simulink model "final_quadruped_040722_zmp"  (R2021a)
settings: Solver=ode15s  StartTime=0.0  StopTime=10  FixedStep=1e-3  RelTol=1e-5  EnableMultiTasking=on
values from neighbouring files (symbols this model uses):
  foot_x = 8    [bipedparameters.m]    (also in fcn.m; finalrobotParameters.m; finalrobotParameters_110522.m; finalrobotParameters_140522.m)
  foot_y = 6    [bipedparameters.m]    (also in fcn.m; finalrobotParameters.m; finalrobotParameters_110522.m; finalrobotParameters_140522.m)
  foot_z = 1    [bipedparameters.m]    (also in fcn.m; finalrobotParameters.m; finalrobotParameters_110522.m; finalrobotParameters_140522.m)
  height_plane = 0.025    [bipedparameters.m]    (also in finalrobotParameters.m; finalrobotParameters_110522.m; finalrobotParameters_140522.m; finalrobotParameters_240522.m)
  kd_ankle = 1000    [bipedparameters.m]    (also in finalrobotParameters_240522.m)
  kd_hip = 1000    [bipedparameters.m]    (also in finalrobotParameters_240522.m)
  kd_knee = 1000    [bipedparameters.m]    (also in finalrobotParameters_240522.m)
  ki_ankle = 1000    [bipedparameters.m]    (also in finalrobotParameters_240522.m)
  ki_hip = 1000    [bipedparameters.m]    (also in finalrobotParameters_240522.m)
  ki_knee = 2000    [bipedparameters.m]    (also in finalrobotParameters_240522.m)
  kp_ankle = 1000    [bipedparameters.m]    (also in finalrobotParameters_240522.m)
  kp_hip = 1000    [bipedparameters.m]    (also in finalrobotParameters_240522.m)
  kp_knee = 2000    [bipedparameters.m]    (also in finalrobotParameters_240522.m)
  lower_leg_length = 10    [bipedparameters.m]    (also in fcn.m; finalrobotParameters.m; finalrobotParameters_110522.m; finalrobotParameters_140522.m)
  plane_x = 25    [bipedparameters.m]    (also in finalrobotParameters.m; finalrobotParameters_110522.m; finalrobotParameters_140522.m; finalrobotParameters_240522.m)
  plane_y = 3    [bipedparameters.m]    (also in finalrobotParameters.m; finalrobotParameters_110522.m; finalrobotParameters_140522.m; finalrobotParameters_240522.m)
  torso_offset_x = -0.5    [bipedparameters.m]    (also in finalrobotParameters.m = 10; finalrobotParameters_110522.m = 10; finalrobotParameters_140522.m = 10; finalrobotParameters_240522.m = 10)
  torso_offset_z = -2    [bipedparameters.m]    (also in finalrobotParameters.m; finalrobotParameters_110522.m; finalrobotParameters_140522.m; finalrobotParameters_240522.m)
  torso_x = 5    [bipedparameters.m]    (also in fcn.m = 25; finalrobotParameters.m = 25; finalrobotParameters_110522.m = 25; finalrobotParameters_140522.m = 25)
  torso_y = 10    [bipedparameters.m]    (also in fcn.m = 16; finalrobotParameters.m = 16; finalrobotParameters_110522.m = 16; finalrobotParameters_140522.m = 16)
  torso_z = 8    [bipedparameters.m]    (also in fcn.m = 10; finalrobotParameters.m = 10; finalrobotParameters_110522.m = 10; finalrobotParameters_140522.m = 10)
  upper_leg_length = 10    [bipedparameters.m]    (also in fcn.m; finalrobotParameters.m; finalrobotParameters_110522.m; finalrobotParameters_140522.m)
undefined symbols (not defined in the file or in its folder): sigbuilder_block, X, Y, Z
libraries: nesl_utility x288, sm_lib x71, pid_lib x20, Contact_Forces_Lib x16, fl_lib x3
(part 8 of 9)

== system final_quadruped_040722_zmp/Model/Right Leg Front /Hip ==
  note: accelerationRFhip
  t2ddhip : Inport
  tddRF_hip : Inport  Port=2
  Gimbal Joint : sm_lib/Joints/Gimbal Joint  JointMode=Normal  SenseConstraintForce=off  SenseConstraintForceX=off  SenseConstraintForceY=off  SenseConstraintForceZ=off  SenseConstraintTorque=off  SenseConstraintTorqueX=off  SenseConstraintTorqueY=off  SenseConstraintTorqueZ=off  SenseTotalForce=off  SenseTotalForceX=off  SenseTotalForceY=off  SenseTotalForceZ=off  SenseTotalTorque=off  SenseTotalTorqueX=off  SenseTotalTorqueY=off  SenseTotalTorqueZ=off  CompositeWrenchDir=FollowerOnBase  CompositeWrenchFrame=BaseFrame  RxEquilibriumPosition=0  RxEquilibriumPositionUnits=deg  RxSpringStiffness=0  RxSpringStiffnessUnits=N*m/deg  RxDampingCoefficient=0  RxDampingCoefficientUnits=N*m/(deg/s)  RxTorqueActuationMode=InputTorque  RxMotionActuationMode=ComputedMotion  RxSensePosition=on  RxSenseVelocity=on  RxSenseAcceleration=on  RxSenseTorqueForce=off  RxSenseLowerLimitTorqueForce=off  RxSenseUpperLimitTorqueForce=off  RxLowerLimitSpecify=off  RxLowerLimitBound=-90  RxLowerLimitBoundUnits=deg  RxLowerLimitStiffness=1e4  RxLowerLimitStiffnessUnits=N*m/deg  RxLowerLimitDamping=10  RxLowerLimitDampingUnits=N*m/(deg/s)  RxLowerLimitTransitionRegionWidth=0.1  RxLowerLimitTransitionRegionWidthUnits=deg  RxUpperLimitSpecify=off  RxUpperLimitBound=90  RxUpperLimitBoundUnits=deg  RxUpperLimitStiffness=1e4  RxUpperLimitStiffnessUnits=N*m/deg  RxUpperLimitDamping=10  RxUpperLimitDampingUnits=N*m/(deg/s)  RxUpperLimitTransitionRegionWidth=0.1  RxUpperLimitTransitionRegionWidthUnits=deg  RxPositionTargetSpecify=off  RxPositionTargetPriority=High  RxPositionTargetValue=0  RxPositionTargetValueUnits=deg  RxVelocityTargetSpecify=off  RxVelocityTargetPriority=High  RxVelocityTargetValue=0  RxVelocityTargetValueUnits=deg/s  RyEquilibriumPosition=0  RyEquilibriumPositionUnits=deg  RySpringStiffness=0  RySpringStiffnessUnits=N*m/deg  RyDampingCoefficient=0  RyDampingCoefficientUnits=N*m/(deg/s)  RyTorqueActuationMode=InputTorque  RyMotionActuationMode=ComputedMotion  RySensePosition=on  RySenseVelocity=on  RySenseAcceleration=on  RySenseTorqueForce=off  RySenseLowerLimitTorqueForce=off  RySenseUpperLimitTorqueForce=off  RyLowerLimitSpecify=off  RyLowerLimitBound=-90  RyLowerLimitBoundUnits=deg  RyLowerLimitStiffness=1e4  RyLowerLimitStiffnessUnits=N*m/deg  RyLowerLimitDamping=10  RyLowerLimitDampingUnits=N*m/(deg/s)  RyLowerLimitTransitionRegionWidth=0.1  RyLowerLimitTransitionRegionWidthUnits=deg  RyUpperLimitSpecify=off  RyUpperLimitBound=90  RyUpperLimitBoundUnits=deg  RyUpperLimitStiffness=1e4  RyUpperLimitStiffnessUnits=N*m/deg  RyUpperLimitDamping=10  RyUpperLimitDampingUnits=N*m/(deg/s)  RyUpperLimitTransitionRegionWidth=0.1  RyUpperLimitTransitionRegionWidthUnits=deg  RyPositionTargetSpecify=off  RyPositionTargetPriority=High  RyPositionTargetValue=0  RyPositionTargetValueUnits=deg  RyVelocityTargetSpecify=off  RyVelocityTargetPriority=High  RyVelocityTargetValue=0  RyVelocityTargetValueUnits=deg/s  RzEquilibriumPosition=0  RzEquilibriumPositionUnits=deg  RzSpringStiffness=0  RzSpringStiffnessUnits=N*m/deg  RzDampingCoefficient=0  RzDampingCoefficientUnits=N*m/(deg/s)  RzTorqueActuationMode=InputTorque  RzMotionActuationMode=ComputedMotion  RzSensePosition=on  RzSenseVelocity=on  RzSenseAcceleration=on  RzSenseTorqueForce=off  RzSenseLowerLimitTorqueForce=off  RzSenseUpperLimitTorqueForce=off  RzLowerLimitSpecify=off  RzLowerLimitBound=-90  RzLowerLimitBoundUnits=deg  RzLowerLimitStiffness=1e4  RzLowerLimitStiffnessUnits=N*m/deg  RzLowerLimitDamping=10  RzLowerLimitDampingUnits=N*m/(deg/s)  RzLowerLimitTransitionRegionWidth=0.1  RzLowerLimitTransitionRegionWidthUnits=deg  RzUpperLimitSpecify=off  RzUpperLimitBound=90  RzUpperLimitBoundUnits=deg  RzUpperLimitStiffness=1e4  RzUpperLimitStiffnessUnits=N*m/deg  RzUpperLimitDamping=10  RzUpperLimitDampingUnits=N*m/(deg/s)  RzUpperLimitTransitionRegionWidth=0.1  RzUpperLimitTransitionRegionWidthUnits=deg  RzPositionTargetSpecify=on  RzPositionTargetPriority=Low  RzPositionTargetValue=-13  RzPositionTargetValueUnits=deg  RzVelocityTargetSpecify=on  RzVelocityTargetPriority=Low  RzVelocityTargetValue=1  RzVelocityTargetValueUnits=deg/s
  MATLAB Function : MATLAB Function  TreatAsAtomicUnit=on
  MATLAB Function1 : MATLAB Function  TreatAsAtomicUnit=on
  MATLAB Function2 : MATLAB Function  TreatAsAtomicUnit=on
  MATLAB Function3 : MATLAB Function  TreatAsAtomicUnit=on
  PID Controller : pid_lib/PID Controller  Controller=PID  Form=Parallel  TimeDomain=Continuous-time  UseExternalTs=off  SampleTime=-1  IntegratorMethod=Forward Euler  FilterMethod=Forward Euler  ControllerParametersSource=internal  P=kp_hip  I=ki_hip  D=kd_hip  UseFilter=on  N=100  TunerSelectOption=Transfer Function Based (PID Tuner App)  InitialConditionSource=internal  InitialConditionForIntegrator=0  InitialConditionForFilter=0  DifferentiatorICPrevScaledInput=0  ExternalReset=none  TrackingMode=off  Kt=1  LimitOutput=off  SatLimitsSource=internal  UpperSaturationLimit=inf  LowerSaturationLimit=-inf  LinearizeAsGain=on  AntiWindupMode=none  Kb=1  POutMin=[]  POutMax=[]  IOutMin=[]  IOutMax=[]  DOutMin=[]  DOutMax=[]  NOutMin=[]  NOutMax=[]  SumOutMin=[]  SumOutMax=[]  SaturationOutMin=[]  SaturationOutMax=[]  PParamMin=[]  PParamMax=[]  IParamMin=[]  IParamMax=[]  DParamMin=[]  DParamMax=[]  NParamMin=[]  NParamMax=[]  KbParamMin=[]  KbParamMax=[]  KtParamMin=[]  KtParamMax=[]  KbOutMin=[]  KbOutMax=[]  KtOutMin=[]  KtOutMax=[]  IntegratorOutMin=[]  IntegratorOutMax=[]  FilterOutMin=[]  FilterOutMax=[]  SumI1OutMin=[]  SumI1OutMax=[]  SumI2OutMin=[]  SumI2OutMax=[]  SumI3OutMin=[]  SumI3OutMax=[]  SumI4OutMin=[]  SumI4OutMax=[]  SumDOutMin=[]  SumDOutMax=[]  DifferentiatorOutMin=[]  DifferentiatorOutMax=[]  FilterDiffOutCoefMin=[]  FilterDiffOutCoefMax=[]  ReciprocalOutMin=[]  ReciprocalOutMax=[]  SumDenOutMin=[]  SumDenOutMax=[]  SumNumOutMin=[]  SumNumOutMax=[]  DivideOutMin=[]  DivideOutMax=[]  UdiffTsProdOutMin=[]  UdiffTsProdOutMax=[]  NTsProdOutMin=[]  NTsProdOutMax=[]  UintegralTsProdOutMin=[]  UintegralTsProdOutMax=[]  UngainTsProdOutMin=[]  UngainTsProdOutMax=[]  IntegratorContinuousStateAttributes=''  IntegratorStateMustResolveToSignalObject=off  IntegratorRTWStateStorageClass=Auto  FilterContinuousStateAttributes=''  FilterStateMustResolveToSignalObject=off  FilterRTWStateStorageClass=Auto  ParallelPVariant=InternalParameters  IdealPVariant=Disabled  IVariant=InternalParameters  DVariant=InternalParameters  IntegratorVariant=Continuous  SatVariant=Disabled  AWVariant=Passthrough  PCopyVariant=Disabled  TRVariant=Disabled  FdbkBlocksVariant=Forward  IdealPFdbkVariant=Disabled  SatFdbkVariant=Disabled  DerivativeFilterVariant=ContFilter  NVariant=InternalParameters  NCopyVariant=Disabled  FilterICVariant=InternalICsFilter  IntegratorICVariant=InternalICs  ExternalResetVariant=Disabled  TRSumVariant=Passthrough  SumFdbkVariant=Disabled  SumVariant=Sum_PID  TsampFilterVariant=InternalTs  TsampNgainVariant=Passthrough  TsampIntegralVariant=Passthrough  ExternalSaturationOutDataTypeStr=Inherit: Same as second input
  PID Controller1 : pid_lib/PID Controller  Controller=PID  Form=Parallel  TimeDomain=Continuous-time  UseExternalTs=off  SampleTime=-1  IntegratorMethod=Forward Euler  FilterMethod=Forward Euler  ControllerParametersSource=internal  P=kp_hip  I=ki_hip  D=kd_hip  UseFilter=on  N=100  TunerSelectOption=Transfer Function Based (PID Tuner App)  InitialConditionSource=internal  InitialConditionForIntegrator=0  InitialConditionForFilter=0  DifferentiatorICPrevScaledInput=0  ExternalReset=none  TrackingMode=off  Kt=1  LimitOutput=off  SatLimitsSource=internal  UpperSaturationLimit=inf  LowerSaturationLimit=-inf  LinearizeAsGain=on  AntiWindupMode=none  Kb=1  POutMin=[]  POutMax=[]  IOutMin=[]  IOutMax=[]  DOutMin=[]  DOutMax=[]  NOutMin=[]  NOutMax=[]  SumOutMin=[]  SumOutMax=[]  SaturationOutMin=[]  SaturationOutMax=[]  PParamMin=[]  PParamMax=[]  IParamMin=[]  IParamMax=[]  DParamMin=[]  DParamMax=[]  NParamMin=[]  NParamMax=[]  KbParamMin=[]  KbParamMax=[]  KtParamMin=[]  KtParamMax=[]  KbOutMin=[]  KbOutMax=[]  KtOutMin=[]  KtOutMax=[]  IntegratorOutMin=[]  IntegratorOutMax=[]  FilterOutMin=[]  FilterOutMax=[]  SumI1OutMin=[]  SumI1OutMax=[]  SumI2OutMin=[]  SumI2OutMax=[]  SumI3OutMin=[]  SumI3OutMax=[]  SumI4OutMin=[]  SumI4OutMax=[]  SumDOutMin=[]  SumDOutMax=[]  DifferentiatorOutMin=[]  DifferentiatorOutMax=[]  FilterDiffOutCoefMin=[]  FilterDiffOutCoefMax=[]  ReciprocalOutMin=[]  ReciprocalOutMax=[]  SumDenOutMin=[]  SumDenOutMax=[]  SumNumOutMin=[]  SumNumOutMax=[]  DivideOutMin=[]  DivideOutMax=[]  UdiffTsProdOutMin=[]  UdiffTsProdOutMax=[]  NTsProdOutMin=[]  NTsProdOutMax=[]  UintegralTsProdOutMin=[]  UintegralTsProdOutMax=[]  UngainTsProdOutMin=[]  UngainTsProdOutMax=[]  IntegratorContinuousStateAttributes=''  IntegratorStateMustResolveToSignalObject=off  IntegratorRTWStateStorageClass=Auto  FilterContinuousStateAttributes=''  FilterStateMustResolveToSignalObject=off  FilterRTWStateStorageClass=Auto  ParallelPVariant=InternalParameters  IdealPVariant=Disabled  IVariant=InternalParameters  DVariant=InternalParameters  IntegratorVariant=Continuous  SatVariant=Disabled  AWVariant=Passthrough  PCopyVariant=Disabled  TRVariant=Disabled  FdbkBlocksVariant=Forward  IdealPFdbkVariant=Disabled  SatFdbkVariant=Disabled  DerivativeFilterVariant=ContFilter  NVariant=InternalParameters  NCopyVariant=Disabled  FilterICVariant=InternalICsFilter  IntegratorICVariant=InternalICs  ExternalResetVariant=Disabled  TRSumVariant=Passthrough  SumFdbkVariant=Disabled  SumVariant=Sum_PID  TsampFilterVariant=InternalTs  TsampNgainVariant=Passthrough  TsampIntegralVariant=Passthrough  ExternalSaturationOutDataTypeStr=Inherit: Same as second input
  PID Controller2 : pid_lib/PID Controller  Controller=PID  Form=Parallel  TimeDomain=Continuous-time  UseExternalTs=off  SampleTime=-1  IntegratorMethod=Forward Euler  FilterMethod=Forward Euler  ControllerParametersSource=internal  P=kp_hip  I=ki_hip  D=kd_hip  UseFilter=on  N=100  TunerSelectOption=Transfer Function Based (PID Tuner App)  InitialConditionSource=internal  InitialConditionForIntegrator=0  InitialConditionForFilter=0  DifferentiatorICPrevScaledInput=0  ExternalReset=none  TrackingMode=off  Kt=1  LimitOutput=off  SatLimitsSource=internal  UpperSaturationLimit=inf  LowerSaturationLimit=-inf  LinearizeAsGain=on  AntiWindupMode=none  Kb=1  POutMin=[]  POutMax=[]  IOutMin=[]  IOutMax=[]  DOutMin=[]  DOutMax=[]  NOutMin=[]  NOutMax=[]  SumOutMin=[]  SumOutMax=[]  SaturationOutMin=[]  SaturationOutMax=[]  PParamMin=[]  PParamMax=[]  IParamMin=[]  IParamMax=[]  DParamMin=[]  DParamMax=[]  NParamMin=[]  NParamMax=[]  KbParamMin=[]  KbParamMax=[]  KtParamMin=[]  KtParamMax=[]  KbOutMin=[]  KbOutMax=[]  KtOutMin=[]  KtOutMax=[]  IntegratorOutMin=[]  IntegratorOutMax=[]  FilterOutMin=[]  FilterOutMax=[]  SumI1OutMin=[]  SumI1OutMax=[]  SumI2OutMin=[]  SumI2OutMax=[]  SumI3OutMin=[]  SumI3OutMax=[]  SumI4OutMin=[]  SumI4OutMax=[]  SumDOutMin=[]  SumDOutMax=[]  DifferentiatorOutMin=[]  DifferentiatorOutMax=[]  FilterDiffOutCoefMin=[]  FilterDiffOutCoefMax=[]  ReciprocalOutMin=[]  ReciprocalOutMax=[]  SumDenOutMin=[]  SumDenOutMax=[]  SumNumOutMin=[]  SumNumOutMax=[]  DivideOutMin=[]  DivideOutMax=[]  UdiffTsProdOutMin=[]  UdiffTsProdOutMax=[]  NTsProdOutMin=[]  NTsProdOutMax=[]  UintegralTsProdOutMin=[]  UintegralTsProdOutMax=[]  UngainTsProdOutMin=[]  UngainTsProdOutMax=[]  IntegratorContinuousStateAttributes=''  IntegratorStateMustResolveToSignalObject=off  IntegratorRTWStateStorageClass=Auto  FilterContinuousStateAttributes=''  FilterStateMustResolveToSignalObject=off  FilterRTWStateStorageClass=Auto  ParallelPVariant=InternalParameters  IdealPVariant=Disabled  IVariant=InternalParameters  DVariant=InternalParameters  IntegratorVariant=Continuous  SatVariant=Disabled  AWVariant=Passthrough  PCopyVariant=Disabled  TRVariant=Disabled  FdbkBlocksVariant=Forward  IdealPFdbkVariant=Disabled  SatFdbkVariant=Disabled  DerivativeFilterVariant=ContFilter  NVariant=InternalParameters  NCopyVariant=Disabled  FilterICVariant=InternalICsFilter  IntegratorICVariant=InternalICs  ExternalResetVariant=Disabled  TRSumVariant=Passthrough  SumFdbkVariant=Disabled  SumVariant=Sum_PID  TsampFilterVariant=InternalTs  TsampNgainVariant=Passthrough  TsampIntegralVariant=Passthrough  ExternalSaturationOutDataTypeStr=Inherit: Same as second input
  PS-Simulink Converter{,2..11} (11 alike) : nesl_utility/PS-Simulink Converter  PhysicalDomain=network_engine_domain  SubClassName=ps_output  LeftPortType=input  RightPortType=output  PseudoPeriodic=off  Frequencies=[]  Unit=inherit  AffineConversion=off
      settings: SourceProductBaseCode=PW,SS
  PS-Simulink Converter1 : nesl_utility/PS-Simulink Converter  PhysicalDomain=network_engine_domain  SubClassName=ps_output  LeftPortType=input  RightPortType=output  PseudoPeriodic=off  Frequencies=[]  Unit=1  AffineConversion=off
      settings: SourceProductBaseCode=PW,SS
  Scope{,1..6} (7 alike) : Scope
  Simulink-PS Converter : nesl_utility/Simulink-PS Converter  PhysicalDomain=network_engine_domain  SubClassName=ps_input  LeftPortType=input  RightPortType=output  PseudoPeriodic=off  Frequencies=[]  NoiseDistribution=none  NoiseParameters=[]  Unit=1  AffineConversion=off  FilteringAndDerivatives=provide  SimscapeFilterOrder=1  InputFilterTimeConstant=0.001  UdotUserProvided=0
      settings: SourceProductBaseCode=PW,SS
  Simulink-PS Converter1 : nesl_utility/Simulink-PS Converter  PhysicalDomain=network_engine_domain  SubClassName=ps_input  LeftPortType=input  RightPortType=output  PseudoPeriodic=off  Frequencies=[]  NoiseDistribution=none  NoiseParameters=[]  Unit=1  AffineConversion=off  FilteringAndDerivatives=provide  SimscapeFilterOrder=1  InputFilterTimeConstant=0.001  UdotUserProvided=0
      settings: SourceProductBaseCode=PW,SS
  Simulink-PS Converter2 : nesl_utility/Simulink-PS Converter  PhysicalDomain=network_engine_domain  SubClassName=ps_input  LeftPortType=input  RightPortType=output  PseudoPeriodic=off  Frequencies=[]  NoiseDistribution=none  NoiseParameters=[]  Unit=1  AffineConversion=off  FilteringAndDerivatives=provide  SimscapeFilterOrder=1  InputFilterTimeConstant=0.001  UdotUserProvided=0
      settings: SourceProductBaseCode=PW,SS
  Sum : Sum  Inputs=|+-
  Sum1 : Sum  Inputs=|+-
  Sum2 : Sum  Inputs=|+-
  Conn1 : PMIOPort  Side=Left
  Conn2 : PMIOPort  Port=2  Side=Right
  qx : PMIOPort  Port=3  Side=Right
  qy : PMIOPort  Port=4  Side=Right
  qz : PMIOPort  Port=5  Side=Right
  Outport2 : Outport
  Outport1 : Outport  Port=2
  Outport : Outport  Port=3
  wires:
  PS-Simulink Converter1/1 -> Sum/2  "speedRFhip"
  Sum/1 -> PID Controller/1, Scope/1
  PID Controller/1 -> Scope1/1, Simulink-PS Converter/1  "torqueRFhip"
  MATLAB Function1/1(hip) -> Outport2/1
  t2ddhip/1 -> Scope2/1
  PS-Simulink Converter/1 -> MATLAB Function/1(qx)
  PS-Simulink Converter4/1 -> MATLAB Function/2(qy)
  PS-Simulink Converter5/1 -> MATLAB Function/3(qz)
  MATLAB Function/1(hip) -> Outport1/1
  PS-Simulink Converter6/1 -> MATLAB Function1/1(wx)
  PS-Simulink Converter7/1 -> MATLAB Function1/2(wy)
  PS-Simulink Converter8/1 -> MATLAB Function1/3(wz)
  tddRF_hip/1 -> MATLAB Function2/1(tddRF)
  PID Controller1/1 -> Simulink-PS Converter1/1, Scope4/1  "torqueRFhip"
  Sum1/1 -> PID Controller1/1, Scope3/1
  MATLAB Function2/1(tddRFx) -> Sum1/1
  PS-Simulink Converter2/1 -> Sum1/2
  MATLAB Function2/3(tddRFz) -> Sum/1
  PID Controller2/1 -> Simulink-PS Converter2/1, Scope6/1  "torqueRFhip"
  Sum2/1 -> PID Controller2/1, Scope5/1
  MATLAB Function2/2(tddRFy) -> Sum2/1
  PS-Simulink Converter9/1 -> Sum2/2
  PS-Simulink Converter10/1 -> MATLAB Function3/1(bx)
  PS-Simulink Converter3/1 -> MATLAB Function3/3(bz)
  PS-Simulink Converter11/1 -> MATLAB Function3/2(by)
  MATLAB Function3/1(hip) -> Outport/1
  connections:
  Conn2/RConn1 -- Gimbal Joint/RConn1
  Conn1/RConn1 -- Gimbal Joint/LConn1
  Gimbal Joint/RConn2 -- qx/RConn1 -- PS-Simulink Converter/LConn1
  PS-Simulink Converter4/LConn1 -- Gimbal Joint/RConn5 -- qy/RConn1
  PS-Simulink Converter5/LConn1 -- Gimbal Joint/RConn8 -- qz/RConn1
  Gimbal Joint/RConn3 -- PS-Simulink Converter2/LConn1 -- PS-Simulink Converter6/LConn1
  PS-Simulink Converter7/LConn1 -- Gimbal Joint/RConn6 -- PS-Simulink Converter9/LConn1
  PS-Simulink Converter8/LConn1 -- Gimbal Joint/RConn9 -- PS-Simulink Converter1/LConn1
  Simulink-PS Converter1/RConn1 -- Gimbal Joint/LConn2
  Simulink-PS Converter2/RConn1 -- Gimbal Joint/LConn3
  Simulink-PS Converter/RConn1 -- Gimbal Joint/LConn4
  Gimbal Joint/RConn4 -- PS-Simulink Converter10/LConn1
  Gimbal Joint/RConn7 -- PS-Simulink Converter11/LConn1
  Gimbal Joint/RConn10 -- PS-Simulink Converter3/LConn1

== system final_quadruped_040722_zmp/Model/Right Leg Front /Knee ==
  note: accelerationRFknee
  note: Meas for knee
  tddRF_knee : Inport
  t2ddknee : Inport  Port=2
  Bus Creator : BusCreator  Inputs=3
  Knee joint : sm_lib/Joints/Revolute Joint  JointMode=Normal  SenseConstraintForce=off  SenseConstraintForceX=off  SenseConstraintForceY=off  SenseConstraintForceZ=off  SenseConstraintTorque=off  SenseConstraintTorqueX=off  SenseConstraintTorqueY=off  SenseConstraintTorqueZ=off  SenseTotalForce=off  SenseTotalForceX=off  SenseTotalForceY=off  SenseTotalForceZ=off  SenseTotalTorque=off  SenseTotalTorqueX=off  SenseTotalTorqueY=off  SenseTotalTorqueZ=off  CompositeWrenchDir=FollowerOnBase  CompositeWrenchFrame=BaseFrame  EquilibriumPosition=0  EquilibriumPositionUnits=deg  SpringStiffness=0  SpringStiffnessUnits=N*m/deg  DampingCoefficient=0  DampingCoefficientUnits=N*m/(deg/s)  TorqueActuationMode=InputTorque  MotionActuationMode=ComputedMotion  SensePosition=on  SenseVelocity=on  SenseAcceleration=on  SenseTorqueForce=off  SenseLowerLimitTorqueForce=off  SenseUpperLimitTorqueForce=off  LowerLimitSpecify=on  LowerLimitBound=0  LowerLimitBoundUnits=deg  LowerLimitStiffness=1e4  LowerLimitStiffnessUnits=N*m/deg  LowerLimitDamping=10  LowerLimitDampingUnits=N*m/(deg/s)  LowerLimitTransitionRegionWidth=0.1  LowerLimitTransitionRegionWidthUnits=deg  UpperLimitSpecify=on  UpperLimitBound=20  UpperLimitBoundUnits=deg  UpperLimitStiffness=1e4  UpperLimitStiffnessUnits=N*m/deg  UpperLimitDamping=10  UpperLimitDampingUnits=N*m/(deg/s)  UpperLimitTransitionRegionWidth=0.1  UpperLimitTransitionRegionWidthUnits=deg  PositionTargetSpecify=on  PositionTargetPriority=Low  PositionTargetValue=28  PositionTargetValueUnits=deg  VelocityTargetSpecify=on  VelocityTargetPriority=Low  VelocityTargetValue=-2  VelocityTargetValueUnits=deg/s
  PID Controller : pid_lib/PID Controller  Controller=PID  Form=Parallel  TimeDomain=Continuous-time  UseExternalTs=off  SampleTime=-1  IntegratorMethod=Forward Euler  FilterMethod=Forward Euler  ControllerParametersSource=internal  P=kp_knee  I=ki_knee  D=kd_knee  UseFilter=on  N=100  TunerSelectOption=Transfer Function Based (PID Tuner App)  InitialConditionSource=internal  InitialConditionForIntegrator=0  InitialConditionForFilter=0  DifferentiatorICPrevScaledInput=0  ExternalReset=none  TrackingMode=off  Kt=1  LimitOutput=off  SatLimitsSource=internal  UpperSaturationLimit=inf  LowerSaturationLimit=-inf  LinearizeAsGain=on  AntiWindupMode=none  Kb=1  POutMin=[]  POutMax=[]  IOutMin=[]  IOutMax=[]  DOutMin=[]  DOutMax=[]  NOutMin=[]  NOutMax=[]  SumOutMin=[]  SumOutMax=[]  SaturationOutMin=[]  SaturationOutMax=[]  PParamMin=[]  PParamMax=[]  IParamMin=[]  IParamMax=[]  DParamMin=[]  DParamMax=[]  NParamMin=[]  NParamMax=[]  KbParamMin=[]  KbParamMax=[]  KtParamMin=[]  KtParamMax=[]  KbOutMin=[]  KbOutMax=[]  KtOutMin=[]  KtOutMax=[]  IntegratorOutMin=[]  IntegratorOutMax=[]  FilterOutMin=[]  FilterOutMax=[]  SumI1OutMin=[]  SumI1OutMax=[]  SumI2OutMin=[]  SumI2OutMax=[]  SumI3OutMin=[]  SumI3OutMax=[]  SumI4OutMin=[]  SumI4OutMax=[]  SumDOutMin=[]  SumDOutMax=[]  DifferentiatorOutMin=[]  DifferentiatorOutMax=[]  FilterDiffOutCoefMin=[]  FilterDiffOutCoefMax=[]  ReciprocalOutMin=[]  ReciprocalOutMax=[]  SumDenOutMin=[]  SumDenOutMax=[]  SumNumOutMin=[]  SumNumOutMax=[]  DivideOutMin=[]  DivideOutMax=[]  UdiffTsProdOutMin=[]  UdiffTsProdOutMax=[]  NTsProdOutMin=[]  NTsProdOutMax=[]  UintegralTsProdOutMin=[]  UintegralTsProdOutMax=[]  UngainTsProdOutMin=[]  UngainTsProdOutMax=[]  IntegratorContinuousStateAttributes=''  IntegratorStateMustResolveToSignalObject=off  IntegratorRTWStateStorageClass=Auto  FilterContinuousStateAttributes=''  FilterStateMustResolveToSignalObject=off  FilterRTWStateStorageClass=Auto  ParallelPVariant=InternalParameters  IdealPVariant=Disabled  IVariant=InternalParameters  DVariant=InternalParameters  IntegratorVariant=Continuous  SatVariant=Disabled  AWVariant=Passthrough  PCopyVariant=Disabled  TRVariant=Disabled  FdbkBlocksVariant=Forward  IdealPFdbkVariant=Disabled  SatFdbkVariant=Disabled  DerivativeFilterVariant=ContFilter  NVariant=InternalParameters  NCopyVariant=Disabled  FilterICVariant=InternalICsFilter  IntegratorICVariant=InternalICs  ExternalResetVariant=Disabled  TRSumVariant=Passthrough  SumFdbkVariant=Disabled  SumVariant=Sum_PID  TsampFilterVariant=InternalTs  TsampNgainVariant=Passthrough  TsampIntegralVariant=Passthrough  ExternalSaturationOutDataTypeStr=Inherit: Same as second input
  PS-Simulink Converter : nesl_utility/PS-Simulink Converter  PhysicalDomain=network_engine_domain  SubClassName=ps_output  LeftPortType=input  RightPortType=output  PseudoPeriodic=off  Frequencies=[]  Unit=inherit  AffineConversion=off
      settings: SourceProductBaseCode=PW,SS
  PS-Simulink Converter1 : nesl_utility/PS-Simulink Converter  PhysicalDomain=network_engine_domain  SubClassName=ps_output  LeftPortType=input  RightPortType=output  PseudoPeriodic=off  Frequencies=[]  Unit=1  AffineConversion=off
      settings: SourceProductBaseCode=PW,SS
  PS-Simulink Converter2 : nesl_utility/PS-Simulink Converter  PhysicalDomain=network_engine_domain  SubClassName=ps_output  LeftPortType=input  RightPortType=output  PseudoPeriodic=off  Frequencies=[]  Unit=inherit  AffineConversion=off
      settings: SourceProductBaseCode=PW,SS
  PS-Simulink Converter3 : nesl_utility/PS-Simulink Converter  PhysicalDomain=network_engine_domain  SubClassName=ps_output  LeftPortType=input  RightPortType=output  PseudoPeriodic=off  Frequencies=[]  Unit=1  AffineConversion=off
      settings: SourceProductBaseCode=PW,SS
  Scope : Scope
  Scope1 : Scope
  Scope2 : Scope
  Simulink-PS Converter : nesl_utility/Simulink-PS Converter  PhysicalDomain=network_engine_domain  SubClassName=ps_input  LeftPortType=input  RightPortType=output  PseudoPeriodic=off  Frequencies=[]  NoiseDistribution=none  NoiseParameters=[]  Unit=1  AffineConversion=off  FilteringAndDerivatives=provide  SimscapeFilterOrder=1  InputFilterTimeConstant=0.001  UdotUserProvided=0
      settings: SourceProductBaseCode=PW,SS
  Sum : Sum  Inputs=|+-
  Conn1 : PMIOPort  Side=Left
  Conn2 : PMIOPort  Port=2  Side=Right
  q : PMIOPort  Port=3  Side=Left
  meas : Outport
  Outport : Outport  Port=2
  Outport2 : Outport  Port=3
  wires:
  Bus Creator/1 -> meas/1
  PS-Simulink Converter3/1 -> Bus Creator/1  "angleRFknee"
  PS-Simulink Converter1/1 -> Outport/1, Bus Creator/2  "speedRFknee"
  Sum/1 -> Scope1/1, PID Controller/1
  PID Controller/1 -> Bus Creator/3, Simulink-PS Converter/1, Scope/1  "torqueRFknee"
  PS-Simulink Converter2/1 -> Outport2/1
  PS-Simulink Converter/1 -> Sum/2
  t2ddknee/1 -> Scope2/1
  tddRF_knee/1 -> Sum/1
  connections:
  Knee joint/RConn2 -- q/RConn1 -- PS-Simulink Converter3/LConn1
  Knee joint/LConn1 -- Conn1/RConn1
  Conn2/RConn1 -- Knee joint/RConn1
  PS-Simulink Converter1/LConn1 -- Knee joint/RConn3 -- PS-Simulink Converter/LConn1
  Simulink-PS Converter/RConn1 -- Knee joint/LConn2
  PS-Simulink Converter2/LConn1 -- Knee joint/RConn4

== system final_quadruped_040722_zmp/Model/Right Leg Front /Subsystem ==
  qaa : Inport
  qhaz : Inport  Port=2
  Qquat : Inport  Port=3
  qka : Inport  Port=4
  td4 : Inport  Port=5
  td5 : Inport  Port=6
  w_torso : Inport  Port=7
  vlinks : Inport  Port=8
  v_torso : Inport  Port=9
  qhax : Inport  Port=10
  qhay : Inport  Port=11
  CMg : Inport  Port=12
  td123 : Inport  Port=13
  MATLAB Function : MATLAB Function  TreatAsAtomicUnit=on
  MATLAB Function1 : MATLAB Function  TreatAsAtomicUnit=on
  MATLAB Function2 : MATLAB Function  TreatAsAtomicUnit=on
  MATLAB Function4 : MATLAB Function  TreatAsAtomicUnit=on
  To Workspace : ToWorkspace  VariableName=h_dotRF  SaveFormat=Timeseries  SampleTime=-1
  To Workspace2 : ToWorkspace  VariableName=ea4g  SaveFormat=Timeseries  SampleTime=-1
  To Workspace4 : ToWorkspace  VariableName=ea5g  SaveFormat=Timeseries  SampleTime=-1
  To Workspace5 : ToWorkspace  VariableName=cma4  SaveFormat=Timeseries  SampleTime=-1
  To Workspace6 : ToWorkspace  VariableName=aa3g  SaveFormat=Timeseries  SampleTime=-1
  To Workspace7 : ToWorkspace  VariableName=aa4g  SaveFormat=Timeseries  SampleTime=-1
  To Workspace8 : ToWorkspace  VariableName=cma5  SaveFormat=Timeseries  SampleTime=-1
  hRF : Outport
  h_dotRF : Outport  Port=2
  Qd5g : Outport  Port=3
  alpRF : Outport  Port=4
  I3 : Outport  Port=5
  I4 : Outport  Port=6
  I5 : Outport  Port=7
  wires:
  MATLAB Function/12(cma3g) -> MATLAB Function1/9(cma3)
  MATLAB Function/8(aa3g) -> MATLAB Function4/6(aa4g), To Workspace6/1, MATLAB Function1/7(aa30g)
  MATLAB Function/9(aa4g) -> MATLAB Function1/12(aa40g), To Workspace7/1, MATLAB Function4/7(ea5g)
  MATLAB Function/4(ea4g) -> MATLAB Function2/7(ea4g), To Workspace2/1, MATLAB Function1/4(ea40g), MATLAB Function4/4(ea4g)
  MATLAB Function/14(cma5g) -> To Workspace8/1, MATLAB Function1/10(cma5)
  MATLAB Function/3(ea3g) -> MATLAB Function2/6(ea3g), MATLAB Function4/3(ea3g), MATLAB Function1/3(ea30g)
  MATLAB Function/13(cma4g) -> To Workspace5/1, MATLAB Function1/8(cma4)
  MATLAB Function/5(ea5g) -> MATLAB Function4/5(aa3g), To Workspace4/1, MATLAB Function1/11(ea50g), MATLAB Function2/8(ea5g)
  MATLAB Function1/1(hRF) -> hRF/1
  qka/1 -> MATLAB Function/6(qka)
  qaa/1 -> MATLAB Function/4(qaa)
  Qquat/1 -> MATLAB Function/5(Qquat)
  qhaz/1 -> MATLAB Function/1(qhaz)
  td123/1 -> MATLAB Function4/10(td123)
  td4/1 -> MATLAB Function4/12(td4)
  td5/1 -> MATLAB Function4/13(td5)
  vlinks/1 -> MATLAB Function4/8(vlinks)
  v_torso/1 -> MATLAB Function4/11(v_torso)
  MATLAB Function1/2(rhoRF) -> MATLAB Function2/12(rhoRF)
  MATLAB Function2/1(h_dotRF) -> To Workspace/1, h_dotRF/1
  MATLAB Function/15(Qd5g) -> Qd5g/1
  w_torso/1 -> MATLAB Function4/9(w_torso)
  qhax/1 -> MATLAB Function/2(qhax)
  qhay/1 -> MATLAB Function/3(qhay)
  MATLAB Function/1(ea1g) -> MATLAB Function1/1(ea10g), MATLAB Function2/1(ea1g), MATLAB Function4/1(ea1g)
  MATLAB Function/2(ea2g) -> MATLAB Function2/2(ea2g), MATLAB Function4/2(ea2g), MATLAB Function1/2(ea20g)
  MATLAB Function/6(aa1g) -> MATLAB Function1/5(aa10g)
  MATLAB Function/7(aa2g) -> MATLAB Function1/6(aa20g)
  MATLAB Function/10(cma1g) -> MATLAB Function1/13(cma1)
  MATLAB Function/11(cma2g) -> MATLAB Function1/14(cma2)
  MATLAB Function4/1(ea_dg1) -> MATLAB Function2/3(ea_dg1)
  MATLAB Function4/2(ea_dg2) -> MATLAB Function2/4(ea_dg2)
  MATLAB Function4/3(ea_dg3) -> MATLAB Function2/5(ea_dg3)
  MATLAB Function4/4(ea_dg4) -> MATLAB Function2/9(ea_dg4)
  MATLAB Function4/5(ea_dg5) -> MATLAB Function2/10(ea_dg5)
  MATLAB Function4/6(rho_dotRF) -> MATLAB Function2/11(rho_dotRF)
  MATLAB Function/16(I1) -> MATLAB Function1/15(I1)
  MATLAB Function/17(I2) -> MATLAB Function1/16(I2)
  MATLAB Function/18(I3) -> I3/1, MATLAB Function1/17(I3)
  MATLAB Function/19(I4) -> I4/1, MATLAB Function1/18(I4)
  MATLAB Function/20(I5) -> MATLAB Function1/19(I5), I5/1
  CMg/1 -> MATLAB Function1/20(CMg)
  MATLAB Function1/3(alpRF) -> alpRF/1

== matlab function final_quadruped_040722_zmp/Subsystem/ RF/MATLAB Function3 ==
  data: b output; bx input; by input; bz input; px input; py input; pz input; p output; vx input; vy input; v output; vz input; ax input; ay input; az input; a output
function [b,p,v,a] = fcn(bx,by,bz,px,py,pz,vx,vy,vz,ax,ay,az)
b=[bx;by;bz];
p=[px;py;pz];
v=[vx;vy;vz];
a=[ax;ay;az];
end

== matlab function final_quadruped_040722_zmp/Model/Left Leg Front /Subsystem/MATLAB Function2 ==
  data: eb1g input; eb2g input; h_dotLF output; eb_dg1 input; eb_dg2 input; eb_dg3 input; eb3g input; eb4g input; eb5g input; eb_dg4 input; eb_dg5 input; rho_dotLF input; rhoLF input
function h_dotLF = fcn( eb1g,eb2g,eb_dg1,eb_dg2,eb_dg3,eb3g, eb4g, eb5g, eb_dg4, eb_dg5, rho_dotLF, rhoLF)
%%
lower_leg_length = 10;
upper_leg_length = 10;
density = 1000;
foot_density=2000;
leg_radius = 0.75;
foot_x = 8;
foot_y = 6;
foot_z = 1;
m_ul=density*leg_radius*leg_radius*upper_leg_length*3.141592653589*0.01*0.01*0.01;
m_ll=density*leg_radius*leg_radius*lower_leg_length*3.141592653589*0.01*0.01*0.01;
m_foot=foot_density*foot_x*foot_y*foot_z*0.000001;
m1=0;
m2=0;
%%
h1_dot=m1*(cross(eb1g,rho_dotLF(:,1,1)))+m1*(cross(eb_dg1,rhoLF(:,1,1)))+m2*(cross(eb1g,rho_dotLF(:,2,1)))+m2*(cross(eb_dg1,rhoLF(:,2,1)))+m_ul*(cross(eb1g,rho_dotLF(:,3,1)))+m_ul*(cross(eb_dg1,rhoLF(:,3,1)))+m_ll*(cross(eb1g,rho_dotLF(:,4,1)))+m_ll*(cross(eb_dg1,rhoLF(:,4,1)))+m_foot*(cross(eb1g,rho_dotLF(:,5,1)))+m_foot*(cross(eb_dg1,rhoLF(:,5,1)));
h2_dot=m2*(cross(eb2g,rho_dotLF(:,2,2)))+m2*(cross(eb_dg2,rhoLF(:,2,2)))+m_ul*(cross(eb2g,rho_dotLF(:,3,2)))+m_ul*(cross(eb_dg2,rhoLF(:,3,2)))+m_ll*(cross(eb2g,rho_dotLF(:,4,2)))+m_ll*(cross(eb_dg2,rhoLF(:,4,2)))+m_foot*(cross(eb2g,rho_dotLF(:,5,2)))+m_foot*(cross(eb_dg2,rhoLF(:,5,2)));
h3_dot=(m_ul*cross(eb3g,rho_dotLF(:,3,3)))+(m_ul*cross(eb_dg3,rhoLF(:,3,3)))+(m_ll*cross(eb3g,rho_dotLF(:,4,3)))+(m_ll*cross(eb_dg3,rhoLF(:,4,3)))+(m_foot*cross(eb3g,rho_dotLF(:,5,3)))+(m_foot*cross(eb_dg3,rhoLF(:,5,3)));
h4_dot=(m_ll*cross(eb4g,rho_dotLF(:,4,4)))+(m_ll*cross(eb_dg4,rhoLF(:,4,4)))+(m_foot*cross(eb4g,rho_dotLF(:,5,4)))+(m_foot*cross(eb_dg4,rhoLF(:,5,4)));
h5_dot=m_foot*(cross(eb5g,rho_dotLF(:,5,5)))+m_foot*(cross(eb_dg5,rhoLF(:,5,5)));

h_dotLF =[h1_dot h2_dot h3_dot h4_dot h5_dot];



end

== matlab function final_quadruped_040722_zmp/Model/Left Leg Front /Subsystem/MATLAB Function4 ==
  data: eb1g input; eb2g input; eb_dg1 output; eb_dg2 output; eb3g input; eb_dg3 output; eb4g input; ab3g input; ab4g input; eb5g input; vlinks input; w_torso input; eb_dg4 output; td123 input; v_torso input; eb_dg5 output; td4 input; td5 input; rho_dotLF output
function [eb_dg1,eb_dg2,eb_dg3,eb_dg4,eb_dg5,rho_dotLF] = fcn(eb1g,eb2g,eb3g,eb4g,ab3g,ab4g, eb5g, vlinks, w_torso, td123, v_torso, td4, td5)
w0=w_torso;
w1=w0*td123(1);
w2=w1*td123(2);
w3=w2+eb3g*td123(3);
w4=w3+eb4g*td4;
w5=w4+eb5g*td5;

%e dot = omega X e
eb_dg1=cross(w1,eb1g);
eb_dg2=cross(w2,eb2g);
eb_dg3=cross(w3,eb3g);
eb_dg4=cross(w4,eb4g);
eb_dg5=cross(w5,eb5g);


vcf=zeros(3,5);
vof=zeros(3,5);
rho_dotLF=zeros(3,5,5);
vcf(:,1)=0;
vcf(:,2)=0;
vcf(:,3)=vlinks(4);
vcf(:,4)=vlinks(5);
vcf(:,5)=vlinks(6);
vof(:,1)=0;
vof(:,2)=0;
vof(:,3)=v_torso;
vof(:,4)=vof(:,3)+cross(w3,ab3g);
vof(:,5)=vof(:,4)+cross(w4,ab4g);
for i=1:5
    for j=1:5
        if j<i
rho_dotLF(:,j,i)=zeros(3,1);
        else
rho_dotLF(:,j,i)=vcf(:,j)-vof(:,i);
        end
    end
end

end

== matlab function final_quadruped_040722_zmp/Model/Right Leg Back/Subsystem/MATLAB Function ==
  data: ec1g output; ec2g output; ec3g output; ec4g output; ec5g output; ac1g output; ac2g output; qhcz input; qhcx input; qhcy input; qac input; Qquat input; qkc input; ac3g output; ac4g output; cmc1g output; cmc2g output; cmc3g output; cmc4g output; cmc5g output; Qd5g output; I1 output; I2 output; I3 output; I4 output; I5 output
function [ec1g,ec2g,ec3g,ec4g,ec5g,ac1g,ac2g,ac3g,ac4g,cmc1g,cmc2g,cmc3g,cmc4g,cmc5g,Qd5g,I1,I2,I3,I4,I5] = fcn(qhcz,qhcx,qhcy,qac,Qquat,qkc)
%%
lower_leg_length = 10;
upper_leg_length = 10;
foot_offset=[-1; 0; 0];

I1l=zeros(3,3);
I2l=zeros(3,3);
I3l=[1.49747e-05 0 0;
    0 1.49747e-05 0;
    0 0 4.9701e-07];
I4l=[1.49747e-05 0 0;
    0 1.49747e-05 0;
    0 0 4.9701e-07];
I5l=[0 0 2.96e-05;
    0 5.2e-05 0;
    0 0 8e-05];
%%
Qd0g=quat2rotm([Qquat(1) Qquat(2) Qquat(3) Qquat(4)]);

%x,y,z are with respect to joint's frame
%z of joint is y of robot
Qd30z=[cos(qhcz) -sin(qhcz) 0;
      sin(qhcz) cos(qhcz) 0;
      0 0 1];
Qd30y=[cos(qhcy) 0 sin(qhcy);
      0 1 0 ;
      -sin(qhcy) 0 cos(qhcy)];
Qd30x=[1 0 0;
      0 cos(qhcx) -sin(qhcx) ;
      0 sin(qhcx) cos(qhcx)];
  
Qd30=Qd30x*Qd30y*Qd30z;
Qd3g=Qd30*Qd0g;
  
Qd43=[cos(qkc) 0 sin(qkc);
      0 1 0 ;
      -sin(qkc) 0 cos(qkc)];
  
Qd54=[1 0 0;
      0 cos(qac) -sin(qac);
      0 sin(qac) cos(qac)];
  
Qd40 = Qd43* Qd30;
Qd50=Qd54*Qd40;
Qd4g=Qd40*Qd0g;
Qd5g=Qd50*Qd0g;

%axis in local frames
ed1l=[1;0;0];
ed2l=[0;1;0];
ed3l=[0;
      0;
      1];
  
ed4l=[0;
      1;
      0];
ed5l=[0;
     0;
     1];
  
%link vector in local frame
ad3l=[0;
      0;
      -upper_leg_length];
   
ad4l=[0;
      0;
      -lower_leg_length];
         
%axis in global frames
ec1g=Qd30x*Qd0g*ed1l;
ec2g=Qd30x*Qd30y*Qd0g*ed2l;
ec3g = Qd30x*Qd30y*Qd30z*Qd0g*ed3l;
ec4g = Qd4g*ed4l;
ec5g = Qd5g*ed5l;

%link vector in global frame
ac1g=0;
ac2g=0;
ac3g = Qd3g*ad3l;
ac4g = Qd4g*ad4l;

%COM distances in base frame
cmc1g=0;
cmc2g=0;
cmc3g=ac3g/2;
cmc4g=ac4g/2;
cmc5g=Qd5g*foot_offset;

%I in global frame
I1=Qd30x*Qd0g*I1l*transpose(Qd30x*Qd0g);
I2=Qd30x*Qd30y*Qd0g*I2l*transpose(Qd30x*Qd30y*Qd0g);
I3=Qd30x*Qd30y*Qd30z*Qd0g*I3l*transpose(Qd30x*Qd30y*Qd30z*Qd0g);
I4=Qd4g*I4l*transpose(Qd4g);
I5=Qd5g*I5l*transpose(Qd5g);



end

== matlab function final_quadruped_040722_zmp/Model/Right Leg Back/Subsystem/MATLAB Function1 ==
  data: ec10g input; ec20g input; ec30g input; ec40g input; ac10g input; ac20g input; ac30g input; cmc4 input; cmc3 input; cmc5 input; ec50g input; ac40g input; hRB output; rhoRB output; cmc1 input; cmc2 input; CMg input; alpRB output; I1 input; I2 input; I3 input; I4 input; I5 input
function [hRB,rhoRB,alpRB] = fcn(ec10g,ec20g,ec30g, ec40g,ac10g,ac20g, ac30g, cmc4, cmc3, cmc5, ec50g, ac40g,cmc1,cmc2, CMg,I1,I2,I3,I4,I5)
%%
lower_leg_length = 10;
upper_leg_length = 10;
density = 1000;
foot_density=2000;
leg_radius = 0.75;
foot_x = 8;
foot_y = 6;
foot_z = 1;
m_ul=density*leg_radius*leg_radius*upper_leg_length*3.141592653589*0.01*0.01*0.01;
m_ll=density*leg_radius*leg_radius*lower_leg_length*3.141592653589*0.01*0.01*0.01;
m_foot=foot_density*foot_x*foot_y*foot_z*0.000001;
m1=0;
m2=0;
%%
scf=zeros(3,5);
sof=zeros(3,5);
rhoRB=zeros(3,5,5);
scf(:,1)=[0;0;0];
scf(:,2)=[0;0;0];
scf(:,3)=cmc3;
scf(:,4)=ac30g+cmc4;
scf(:,5)=ac30g+ac40g+cmc5;
sof(:,1)=[0;0;0];
sof(:,2)=[0;0;0];
sof(:,3)=[0;0;0];
sof(:,4)=ac30g;
sof(:,5)=ac30g+ac40g;
for i=1:5
    for j=1:5
        if j<i
rhoRB(:,j,i)=zeros(3,1);
        else
rhoRB(:,j,i)=scf(:,j)-sof(:,i);
        end
    end
end

c5=cmc5-CMg;
c4=cmc4-CMg;
c3=cmc3-CMg;
c2=cmc2-CMg;
c1=cmc1-CMg;

h1=m1*(cross(ec10g,rhoRB(:,1,1)))+m2*(cross(ec10g,rhoRB(:,2,1)))+m_ul*(cross(ec10g,rhoRB(:,3,1)))+m_ll*(cross(ec10g,rhoRB(:,4,1)))+m_foot*(cross(ec10g,rhoRB(:,5,1)));
h2=m2*(cross(ec20g,rhoRB(:,2,2)))+m_ul*(cross(ec20g,rhoRB(:,3,2)))+m_ll*(cross(ec20g,rhoRB(:,4,2)))+m_foot*(cross(ec20g,rhoRB(:,5,2)));
h3=(m_ul*cross(ec30g,rhoRB(:,3,3)))+(m_ll*cross(ec30g,rhoRB(:,4,3)))+(m_foot*cross(ec30g,rhoRB(:,5,3)));
h4=(m_ll*cross(ec40g,rhoRB(:,4,4)))+(m_foot*cross(ec40g,rhoRB(:,5,4)));
h5=m_foot*(cross(ec50g,rhoRB(:,5,5)));

hRB =[h1 h2 h3 h4 h5];

alp1=skewsymmetric(c1)*m1*cross(ec10g,rhoRB(:,1,1))+skewsymmetric(c2)*m2*cross(ec10g,rhoRB(:,2,1))+skewsymmetric(c3)*m_ul*cross(ec10g,rhoRB(:,3,1))+skewsymmetric(c4)*m_ll*cross(ec10g,rhoRB(:,4,1))+skewsymmetric(c5)*m_foot*cross(ec10g,rhoRB(:,5,1))+(I1+I2+I3+I4+I5)*ec10g;
alp2=skewsymmetric(c2)*m2*(cross(ec20g,rhoRB(:,2,2)))+skewsymmetric(c3)*m_ul*(cross(ec20g,rhoRB(:,3,2)))+skewsymmetric(c4)*m_ll*(cross(ec20g,rhoRB(:,4,2)))+skewsymmetric(c5)*m_foot*(cross(ec20g,rhoRB(:,5,2)));+(I2+I3+I4+I5)*ec20g;
alp3=skewsymmetric(c3)*m_ul*cross(ec30g,rhoRB(:,3,3))+skewsymmetric(c4)*m_ll*cross(ec30g,rhoRB(:,4,3))+skewsymmetric(c5)*m_foot*cross(ec30g,rhoRB(:,5,3))+(I3+I4+I5)*ec30g;
alp4=skewsymmetric(c4)*m_ll*cross(ec40g,rhoRB(:,4,4))+skewsymmetric(c5)*m_foot*cross(ec40g,rhoRB(:,5,4))+(I4+I5)*ec40g;
alp5=skewsymmetric(c5)*m_foot*cross(ec50g,rhoRB(:,5,5))+I5*ec50g;

alpRB=[alp1 alp2 alp3 alp4 alp5];



end

== matlab function final_quadruped_040722_zmp/Model/Right Leg Back/Subsystem/MATLAB Function2 ==
  data: ec1g input; ec2g input; h_dotRB output; ec_dg1 input; ec_dg2 input; ec_dg3 input; ec3g input; ec4g input; ec5g input; ec_dg4 input; ec_dg5 input; rho_dotRB input; rhoRB input
function h_dotRB = fcn( ec1g,ec2g,ec_dg1,ec_dg2,ec_dg3,ec3g, ec4g, ec5g, ec_dg4, ec_dg5, rho_dotRB, rhoRB)
%%
lower_leg_length = 10;
upper_leg_length = 10;
density = 1000;
foot_density=2000;
leg_radius = 0.75;
foot_x = 8;
foot_y = 6;
foot_z = 1;
m_ul=density*leg_radius*leg_radius*upper_leg_length*3.141592653589*0.01*0.01*0.01;
m_ll=density*leg_radius*leg_radius*lower_leg_length*3.141592653589*0.01*0.01*0.01;
m_foot=foot_density*foot_x*foot_y*foot_z*0.000001;
m1=0;
m2=0;
%%
h1_dot=m1*(cross(ec1g,rho_dotRB(:,1,1)))+m1*(cross(ec_dg1,rhoRB(:,1,1)))+m2*(cross(ec1g,rho_dotRB(:,2,1)))+m2*(cross(ec_dg1,rhoRB(:,2,1)))+m_ul*(cross(ec1g,rho_dotRB(:,3,1)))+m_ul*(cross(ec_dg1,rhoRB(:,3,1)))+m_ll*(cross(ec1g,rho_dotRB(:,4,1)))+m_ll*(cross(ec_dg1,rhoRB(:,4,1)))+m_foot*(cross(ec1g,rho_dotRB(:,5,1)))+m_foot*(cross(ec_dg1,rhoRB(:,5,1)));
h2_dot=m2*(cross(ec2g,rho_dotRB(:,2,2)))+m2*(cross(ec_dg2,rhoRB(:,2,2)))+m_ul*(cross(ec2g,rho_dotRB(:,3,2)))+m_ul*(cross(ec_dg2,rhoRB(:,3,2)))+m_ll*(cross(ec2g,rho_dotRB(:,4,2)))+m_ll*(cross(ec_dg2,rhoRB(:,4,2)))+m_foot*(cross(ec2g,rho_dotRB(:,5,2)))+m_foot*(cross(ec_dg2,rhoRB(:,5,2)));
h3_dot=(m_ul*cross(ec3g,rho_dotRB(:,3,3)))+(m_ul*cross(ec_dg3,rhoRB(:,3,3)))+(m_ll*cross(ec3g,rho_dotRB(:,4,3)))+(m_ll*cross(ec_dg3,rhoRB(:,4,3)))+(m_foot*cross(ec3g,rho_dotRB(:,5,3)))+(m_foot*cross(ec_dg3,rhoRB(:,5,3)));
h4_dot=(m_ll*cross(ec4g,rho_dotRB(:,4,4)))+(m_ll*cross(ec_dg4,rhoRB(:,4,4)))+(m_foot*cross(ec4g,rho_dotRB(:,5,4)))+(m_foot*cross(ec_dg4,rhoRB(:,5,4)));
h5_dot=m_foot*(cross(ec5g,rho_dotRB(:,5,5)))+m_foot*(cross(ec_dg5,rhoRB(:,5,5)));

h_dotRB =[h1_dot h2_dot h3_dot h4_dot h5_dot];



end

== matlab function final_quadruped_040722_zmp/Model/Right Leg Back/Subsystem/MATLAB Function4 ==
  data: ec1g input; ec2g input; ec_dg1 output; ec_dg2 output; ec3g input; ec_dg3 output; ec4g input; ac3g input; ac4g input; ec5g input; vlinks input; w_torso input; ec_dg4 output; td123 input; v_torso input; ec_dg5 output; td4 input; td5 input; rho_dotRB output
function [ec_dg1,ec_dg2,ec_dg3,ec_dg4,ec_dg5,rho_dotRB] = fcn(ec1g,ec2g,ec3g,ec4g,ac3g,ac4g, ec5g, vlinks, w_torso, td123, v_torso, td4, td5)
w0=w_torso;
w1=w0*td123(1);
w2=w1*td123(2);
w3=w2+ec3g*td123(3);
w4=w3+ec4g*td4;
w5=w4+ec5g*td5;

%e dot = omega X e
ec_dg1=cross(w1,ec1g);
ec_dg2=cross(w2,ec2g);
ec_dg3=cross(w3,ec3g);
ec_dg4=cross(w4,ec4g);
ec_dg5=cross(w5,ec5g);


vcf=zeros(3,5);
vof=zeros(3,5);
rho_dotRB=zeros(3,5,5);
vcf(:,1)=0;
vcf(:,2)=0;
vcf(:,3)=vlinks(7);
vcf(:,4)=vlinks(8);
vcf(:,5)=vlinks(9);
vof(:,1)=0;
vof(:,2)=0;
vof(:,3)=v_torso;
vof(:,4)=vof(:,3)+cross(w3,ac3g);
vof(:,5)=vof(:,4)+cross(w4,ac4g);
for i=1:5
    for j=1:5
        if j<i
rho_dotRB(:,j,i)=zeros(3,1);
        else
rho_dotRB(:,j,i)=vcf(:,j)-vof(:,i);
        end
    end
end

end

== matlab function final_quadruped_040722_zmp/Model/Left Leg Back/Subsystem/MATLAB Function ==
  data: ed1g output; ed2g output; ed3g output; ed4g output; ed5g output; ad1g output; ad2g output; qhdz input; qhdx input; qhdy input; qad input; Qquat input; qkd input; ad3g output; ad4g output; cmd1g output; cmd2g output; cmd3g output; cmd4g output; cmd5g output; Qd5g output; I1 output; I2 output; I3 output; I4 output; I5 output
function [ed1g,ed2g,ed3g,ed4g,ed5g,ad1g,ad2g,ad3g,ad4g,cmd1g,cmd2g,cmd3g,cmd4g,cmd5g,Qd5g,I1,I2,I3,I4,I5] = fcn(qhdz,qhdx,qhdy,qad,Qquat,qkd)
%%
lower_leg_length = 10;
upper_leg_length = 10;
foot_offset=[-1; 0; 0];

I1l=zeros(3,3);
I2l=zeros(3,3);
I3l=[1.49747e-05 0 0;
    0 1.49747e-05 0;
    0 0 4.9701e-07];
I4l=[1.49747e-05 0 0;
    0 1.49747e-05 0;
    0 0 4.9701e-07];
I5l=[0 0 2.96e-05;
    0 5.2e-05 0;
    0 0 8e-05];

%%
Qd0g=quat2rotm([Qquat(1) Qquat(2) Qquat(3) Qquat(4)]);

%x,y,z are with respect to joint's frame
%z of joint is y of robot
Qd30z=[cos(qhdz) -sin(qhdz) 0;
      sin(qhdz) cos(qhdz) 0;
      0 0 1];
Qd30y=[cos(qhdy) 0 sin(qhdy);
      0 1 0 ;
      -sin(qhdy) 0 cos(qhdy)];
Qd30x=[1 0 0;
      0 cos(qhdx) -sin(qhdx) ;
      0 sin(qhdx) cos(qhdx)];
  
Qd30=Qd30x*Qd30y*Qd30z;
Qd3g=Qd30*Qd0g; 

  
Qd43=[cos(qkd) 0 sin(qkd);
      0 1 0 ;
      -sin(qkd) 0 cos(qkd)];
  
Qd54=[1 0 0;
      0 cos(qad) -sin(qad);
      0 sin(qad) cos(qad)];
  
Qd40 = Qd43* Qd30;
Qd50=Qd54*Qd40;
Qd4g=Qd40*Qd0g;
Qd5g=Qd50*Qd0g;

%axis in local frames
ed1l=[1;0;0];
ed2l=[0;1;0];
ed3l=[0;
      0;
      1];
  
ed4l=[0;
      1;
      0];
ed5l=[0;
     0;
     1];
  
%link vector in local frame
ad3l=[0;
      0;
      -upper_leg_length];
   
ad4l=[0;
      0;
      -lower_leg_length];
         
%axis in global frames
ed1g=Qd30x*Qd0g*ed1l;
ed2g=Qd30x*Qd30y*Qd0g*ed2l;
ed3g =Qd30x*Qd30y*Qd30z*Qd0g*ed3l;
ed4g = Qd4g*ed4l;
ed5g = Qd5g*ed5l;

%link vector in global frame
ad1g=0;
ad2g=0;
ad3g = Qd3g*ad3l;
ad4g = Qd4g*ad4l;

%COM distances in base frame
cmd1g=0;
cmd2g=0;
cmd3g=ad3g/2;
cmd4g=ad4g/2;
cmd5g=Qd5g*foot_offset;


%I in global frame
I1=Qd30x*Qd0g*I1l*transpose(Qd30x*Qd0g);
I2=Qd30x*Qd30y*Qd0g*I2l*transpose(Qd30x*Qd30y*Qd0g);
I3=Qd30x*Qd30y*Qd30z*Qd0g*I3l*transpose(Qd30x*Qd30y*Qd30z*Qd0g);
I4=Qd4g*I4l*transpose(Qd4g);
I5=Qd5g*I5l*transpose(Qd5g);


end

== matlab function final_quadruped_040722_zmp/Model/Left Leg Back/Subsystem/MATLAB Function1 ==
  data: ed10g input; ed20g input; ed30g input; ed40g input; ad10g input; ad20g input; ad30g input; cmd4 input; cmd3 input; cmd5 input; ed50g input; ad40g input; hLB output; rhoLB output; cmd1 input; CMg input; cmd2 input; alpLB output; I1 input; I2 input; I3 input; I4 input; I5 input
function [hLB,rhoLB,alpLB] = fcn(ed10g,ed20g,ed30g, ed40g,ad10g,ad20g, ad30g, cmd4, cmd3, cmd5, ed50g, ad40g,cmd1,CMg, cmd2,I1,I2,I3,I4,I5)
%%
lower_leg_length = 10;
upper_leg_length = 10;
density = 1000;
foot_density=2000;
leg_radius = 0.75;
foot_x = 8;
foot_y = 6;
foot_z = 1;
m_ul=density*leg_radius*leg_radius*upper_leg_length*3.141592653589*0.01*0.01*0.01;
m_ll=density*leg_radius*leg_radius*lower_leg_length*3.141592653589*0.01*0.01*0.01;
m_foot=foot_density*foot_x*foot_y*foot_z*0.000001;
m1=0;
m2=0;
%%
scf=zeros(3,5);
sof=zeros(3,5);
rhoLB=zeros(3,5,5);
scf(:,1)=[0;0;0];
scf(:,2)=[0;0;0];
scf(:,3)=cmd3;
scf(:,4)=ad30g+cmd4;
scf(:,5)=ad30g+ad40g+cmd5;
sof(:,1)=[0;0;0];
sof(:,2)=[0;0;0];
sof(:,3)=[0;0;0];
sof(:,4)=ad30g;
sof(:,5)=ad30g+ad40g;
for i=1:5
    for j=1:5
        if j<i
rhoLB(:,j,i)=zeros(3,1);
        else
rhoLB(:,j,i)=scf(:,j)-sof(:,i);
        end
    end
end

c5=cmd5-CMg;
c4=cmd4-CMg;
c3=cmd3-CMg;
c2=cmd2-CMg;
c1=cmd1-CMg;

h1=m1*(cross(ed10g,rhoLB(:,1,1)))+m2*(cross(ed10g,rhoLB(:,2,1)))+m_ul*(cross(ed10g,rhoLB(:,3,1)))+m_ll*(cross(ed10g,rhoLB(:,4,1)))+m_foot*(cross(ed10g,rhoLB(:,5,1)));
h2=m2*(cross(ed20g,rhoLB(:,2,2)))+m_ul*(cross(ed20g,rhoLB(:,3,2)))+m_ll*(cross(ed20g,rhoLB(:,4,2)))+m_foot*(cross(ed20g,rhoLB(:,5,2)));
h3=(m_ul*cross(ed30g,rhoLB(:,3,3)))+(m_ll*cross(ed30g,rhoLB(:,4,3)))+(m_foot*cross(ed30g,rhoLB(:,5,3)));
h4=(m_ll*cross(ed40g,rhoLB(:,4,4)))+(m_foot*cross(ed40g,rhoLB(:,5,4)));
h5=m_foot*(cross(ed50g,rhoLB(:,5,5)));

hLB =[h1 h2 h3 h4 h5];

alp1=skewsymmetric(c1)*m1*cross(ed10g,rhoLB(:,1,1))+skewsymmetric(c2)*m2*cross(ed10g,rhoLB(:,2,1))+skewsymmetric(c3)*m_ul*cross(ed10g,rhoLB(:,3,1))+skewsymmetric(c4)*m_ll*cross(ed10g,rhoLB(:,4,1))+skewsymmetric(c5)*m_foot*cross(ed10g,rhoLB(:,5,1))+(I1+I2+I3+I4+I5)*ed10g;
alp2=skewsymmetric(c2)*m2*(cross(ed20g,rhoLB(:,2,2)))+skewsymmetric(c3)*m_ul*(cross(ed20g,rhoLB(:,3,2)))+skewsymmetric(c4)*m_ll*(cross(ed20g,rhoLB(:,4,2)))+skewsymmetric(c5)*m_foot*(cross(ed20g,rhoLB(:,5,2)))+(I2+I3+I4+I5)*ed20g;
alp3=skewsymmetric(c3)*m_ul*cross(ed30g,rhoLB(:,3,3))+skewsymmetric(c4)*m_ll*cross(ed30g,rhoLB(:,4,3))+skewsymmetric(c5)*m_foot*cross(ed30g,rhoLB(:,5,3))+(I3+I4+I5)*ed30g;
alp4=skewsymmetric(c4)*m_ll*cross(ed40g,rhoLB(:,4,4))+skewsymmetric(c5)*m_foot*cross(ed40g,rhoLB(:,5,4))+(I4+I5)*ed40g;
alp5=skewsymmetric(c5)*m_foot*cross(ed50g,rhoLB(:,5,5))+I5*ed50g;

alpLB=[alp1 alp2 alp3 alp4 alp5];



end
